simulink model "resonance_loop2"  (R2022a)
settings: Solver=VariableStepAuto  StartTime=0.0  StopTime=5  MaxStep=1e-3  RelTol=1e-3
undefined symbols (not defined in the file): i
libraries: resonance_lib x2
settings Model: Creator=tstef  LastModifiedBy=tstef

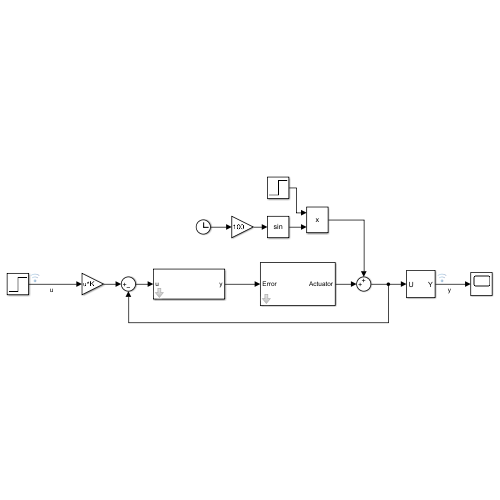
[thumbnail: Simulink's stored preview of the top-level diagram]
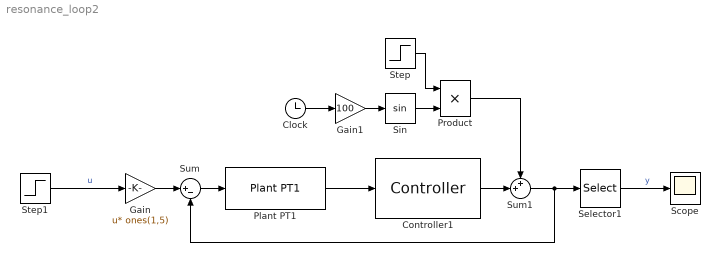
== system resonance_loop2 ==
  Clock : Clock
  Controller1 : resonance_lib/Controller  k_P=43  k_I=10  k_R=95-390*i  k_Ra=950  k_Rb=-3.9e5  k_PIRA=9.3e3  k_PIRAp=-210  k_PIRAz=21  k_ILC=930  T1=0  T1p=-210  T1z=-21  w0=100  zeta=0.05
  Gain : Gain  Gain=ones(1,5)  Multiplication=Matrix(u*K)
  Gain1 : Gain  Gain=100
  Plant PT1 : resonance_lib/Plants/Plant PT1  p=1
  Product : Product
  Scope : Scope
  Selector1 : Selector  NumberOfDimensions=2  InputPortWidth=3  IndexOptions=Select all,Index vector (dialog)  Indices=[1 3],[1 2 3 5]  OutputSizes=1,1
  Sin : Trigonometry
  Step : Step  Time=3  SampleTime=0
  Step1 : Step  Time=0.5  SampleTime=0
  Sum : Sum  Inputs=|+-
  Sum1 : Sum  Inputs=++|
  wires:
  Clock/1 -> Gain1/1
  Sin/1 -> Product/2
  Gain1/1 -> Sin/1
  Step/1 -> Product/1
  Gain/1 -> Sum/1
  Product/1 -> Sum1/1
  Step1/1 -> Gain/1  "u"
  Plant PT1/1 -> Controller1/1
  Sum/1 -> Plant PT1/1
  Sum1/1 -> Sum/2, Selector1/1
  Controller1/1 -> Sum1/2
  Selector1/1 -> Scope/1  "y"
